simulink model "final_fuzzy"  (Simulink 10.1)
settings: Solver=ode45  StartTime=0  StopTime=1  RelTol=1e-3  EnableMultiTasking=on
libraries: powerlib x29, powerlib_extras x6, simulink x2, fuzblock x1
settings Model: Creator=kuldeep  LastModifiedBy=vardh
settings DataIOCC: LimitDataPoints=on  SignalLoggingSaveFormat=ModelDataLogs
settings OptimizationCC: ExpressionDepthLimit=2147483647
settings DebuggingCC: SolverPrmCheckMsg=warning  FcnCallInpInsideContextMsg=warning  StateNameClashWarn=warning
settings GRTTargetCC: CombineOutputUpdateFcns=on  GRTInterface=off
settings SimscapeCC: SimscapeNormalizeSystem=off

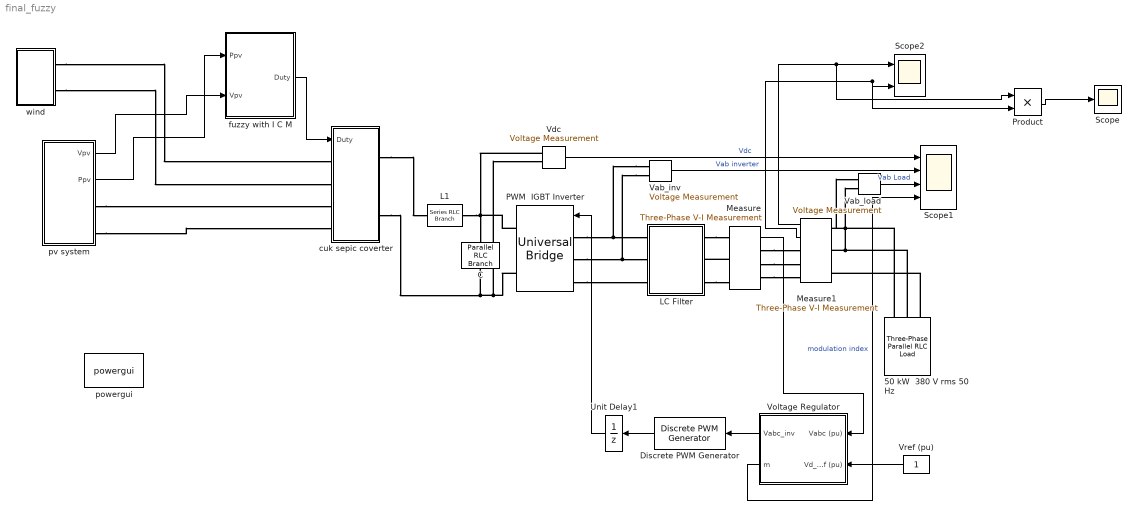
== system final_fuzzy ==
  50 kW  380 V rms 50 Hz : powerlib/Elements/Three-Phase Parallel RLC Load  LConnTagsString=A|B|C  Configuration=Y (grounded)  NominalVoltage=300  Vabc=[1e3 1e3 1e3]  Vabcp=[1e3 1e3 1e3]  NominalFrequency=50  UnbalancedPower=off  ActivePower=30e3  InductivePower=0  CapacitivePower=0  Pabc=[10e3 9e3 11e3]  QLabc=[100 90 110]  QCabc=[100 90 110]  Pabcp=[10e3 9e3 11e3]  QLabcp=[100 90 110]  QCabcp=[100 90 110]  Measurements=None  LoadType=constant Z
  C : powerlib/Elements/Parallel RLC Branch  LConnTagsString=a  RConnTagsString=__new0  BranchType=C  Resistance=inf  Inductance=inf  SetiL0=off  InitialCurrent=0  Capacitance=5000e-06  Setx0=off  InitialVoltage=0  Measurements=None
  Discrete PWM Generator : powerlib_extras/Discrete  Control Blocks/Discrete PWM Generator  GeneratorMode="3-arm  bridge (6 pulses)"  Fc=2000  Ts=3e-5  Internal=off  mIndex=0.4  Freq=60  Phase=0
      settings: SourceProductBaseCode=PS
  L1 : powerlib/Elements/Series RLC Branch  LConnTagsString=__new0  RConnTagsString=__new0  BranchType=L  Resistance=1.0  Inductance=200e-6  SetiL0=off  InitialCurrent=0  Capacitance=1.0  Setx0=off  InitialVoltage=0  Measurements=None
  LC Filter : Subsystem
  Measure : powerlib/Measurements/Three-Phase V-I Measurement  VoltageMeasurement=phase-to-ground  SetLabelV=off  LabelV=V1  Vpu=on  VpuLL=off  CurrentMeasurement=no  SetLabelI=off  LabelI=I1  Ipu=off  Pbase=1e3  Vbase=380  OutputType=Magnitude  PhasorSimulation=off  PSBequivalent=0
  Measure1 : powerlib/Measurements/Three-Phase V-I Measurement  VoltageMeasurement=phase-to-phase  SetLabelV=off  LabelV=V1  Vpu=off  VpuLL=off  CurrentMeasurement=yes  SetLabelI=off  LabelI=I1  Ipu=off  Pbase=1e3  Vbase=380  OutputType=Magnitude  PhasorSimulation=off  PSBequivalent=0
  PWM  IGBT Inverter : powerlib/Power Electronics/Universal Bridge  Arms=3  SnubberResistance=5000  SnubberCapacitance=inf  Device=IGBT / Diodes  Ron=1e-3  Lon=0  ForwardVoltages="[  0.0  0.0  ]"  ForwardVoltage=.8  GTOparameters=[ 1e-6 ,1e-6 ]  IGBTparameters=[ 1e-6 , 2e-6 ]  Measurements=Device currents  Measurements_2=None  converterType=Rectifier
  Product : Product  RndMeth=Zero
  Scope : Scope
  Scope1 : Scope  NumInputPorts=4
  Scope2 : Scope  NumInputPorts=2
  Unit Delay1 : UnitDelay  SampleTime=3e-5  HasFrameUpgradeWarning=on
  Vab_inv : powerlib/Measurements/Voltage Measurement  Tag=PoWeRsYsTeMmEaSuReMeNt  PhasorSimulation=off  OutputType=Magnitude  PSBequivalent=0
  Vab_load : powerlib/Measurements/Voltage Measurement  Tag=PoWeRsYsTeMmEaSuReMeNt  PhasorSimulation=off  OutputType=Magnitude  PSBequivalent=0
  Vdc : powerlib/Measurements/Voltage Measurement  Tag=PoWeRsYsTeMmEaSuReMeNt  PhasorSimulation=off  OutputType=Magnitude  PSBequivalent=0
  Voltage Regulator : Subsystem  mask(Voltage Regulator){Kp=0.4, Ki=500, Ts=3e-5}
      mask prompts: Kp "Proportional gain  Kp:"; Ki "Integral gain Ki:"; Ts "Sample time (s) :"
  "Vref (pu) " : Constant
  cuk sepic coverter : Subsystem
  "fuzzy with I C M " : Subsystem
  powergui : powerlib/powergui  Priority=1  SimulationMode=Discrete  SampleTime=3e-5  frequency=60  Iterations=50  frequencyindice=50  Pbase=100e6  ErrMax=1e-4  UnitsV=kV  UnitsW=MW  buscounter=0  FunctionMessages=off  echomessages=off  EnableUseOfTLC=off  CurrentSourceSwitches=off  DisableSnubberDevices=off  DisableRonSwitches=off  DisableVfSwitches=off  DisplayEquations=off  AutomaticDiscreteSolvers=off  SolverType=Tustin  Interpol=off  ExternalGateDelay=off  methode=off  Ts=100  x0status=blocks  SPID=off  SwTol=0  HookPort=off  NonlinearTolerance=1e-4  nMaxIteration=100  ContinueOnMaxIteration=off  RestoreLinks=warning  ResistiveCurrentMeasurement=off  Frange=[0:2:500]  Ylog=off  Xlog=on  ShowGrid=off  save=off  variable=ZData  structure=ScopeData12  ZoomFFT=off  StartTime=5.86  cycles=1  DisplayStyle=1  fundamental=50  FreqAxis=off  MaxFrequency=1000  frequencyindicesteady=1  RmsSteady=1  display=off
  pv system : Subsystem
  "wind " : Subsystem
  wires:
  pv system/2(Ppv) -> "fuzzy with I C M "/1(Ppv)
  pv system/1(Vpv) -> "fuzzy with I C M "/2(Vpv)
  "fuzzy with I C M "/1(Duty) -> cuk sepic coverter/1(Duty)
  "Vref (pu) "/1 -> Voltage Regulator/2(Vd_ref (pu))
  Discrete PWM Generator/1 -> Unit Delay1/1
  Voltage Regulator/1(Vabc_inv) -> Discrete PWM Generator/1
  Voltage Regulator/2(m) -> Scope1/4  "modulation index"
  Vdc/1 -> Scope1/1  "Vdc"
  Vab_load/1 -> Scope1/3  "Vab Load"
  Vab_inv/1 -> Scope1/2  "Vab inverter"
  Unit Delay1/1 -> PWM  IGBT Inverter/1
  Measure1/1 -> Scope2/1, Product/1
  Measure1/2 -> Scope2/2, Product/2
  Measure/1 -> Voltage Regulator/1(Vabc (pu))
  Product/1 -> Scope/1
  connections:
  pv system/RConn1 -- cuk sepic coverter/LConn3
  pv system/RConn2 -- cuk sepic coverter/LConn4
  "wind "/RConn1 -- cuk sepic coverter/LConn1
  "wind "/RConn2 -- cuk sepic coverter/LConn2
  PWM  IGBT Inverter/RConn2 -- Vdc/LConn2 -- C/RConn1 -- cuk sepic coverter/RConn2
  PWM  IGBT Inverter/RConn1 -- Vdc/LConn1 -- C/LConn1 -- L1/RConn1
  Vab_inv/LConn2 -- PWM  IGBT Inverter/LConn2 -- LC Filter/LConn2
  Vab_inv/LConn1 -- PWM  IGBT Inverter/LConn1 -- LC Filter/LConn1
  LC Filter/RConn1 -- Measure/LConn1
  PWM  IGBT Inverter/LConn3 -- LC Filter/LConn3
  LC Filter/RConn3 -- Measure/LConn3
  Measure/LConn2 -- LC Filter/RConn2
  cuk sepic coverter/RConn1 -- L1/LConn1
  50 kW  380 V rms 50 Hz/LConn1 -- Vab_load/LConn1 -- Measure1/LConn1
  50 kW  380 V rms 50 Hz/LConn2 -- Measure1/LConn2 -- Vab_load/LConn2
  50 kW  380 V rms 50 Hz/LConn3 -- Measure1/LConn3
  Measure/RConn1 -- Measure1/RConn1
  Measure/RConn2 -- Measure1/RConn2
  Measure/RConn3 -- Measure1/RConn3

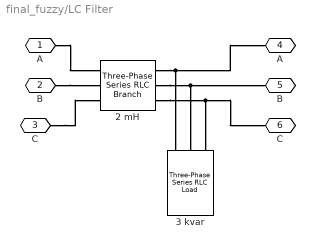
== system final_fuzzy/LC Filter ==
  "2 mH " : powerlib/Elements/Three-Phase Series RLC Branch  LConnTagsString=A|B|C  RConnTagsString=A|B|C  BranchType=L  Resistance=0  Inductance=4e-3  Capacitance=inf  Measurements=None
  3 kvar : powerlib/Elements/Three-Phase Series RLC Load  LConnTagsString=A|B|C  Configuration=Y (grounded)  NominalVoltage=380  Vabc=[1e3 1e3 1e3]  Vabcp=[1e3 1e3 1e3]  NominalFrequency=50  UnbalancedPower=off  ActivePower=0  InductivePower=0  CapacitivePower=3e-6  Pabc=[10e3 9e3 11e3]  QLabc=[100 90 110]  QCabc=[100 90 110]  Pabcp=[10e3 9e3 11e3]  QLabcp=[100 90 110]  QCabcp=[100 90 110]  Measurements=None  LoadType=constant Z
  A : PMIOPort  Side=Left
  B : PMIOPort  Port=2  Side=Left
  C : PMIOPort  Port=3  Side=Left
  "A " : PMIOPort  Port=4  Side=Right
  "B " : PMIOPort  Port=5  Side=Right
  "C " : PMIOPort  Port=6  Side=Right
  connections:
  B/RConn1 -- "2 mH "/LConn2
  A/RConn1 -- "2 mH "/LConn1
  C/RConn1 -- "2 mH "/LConn3
  "2 mH "/RConn1 -- "A "/RConn1 -- 3 kvar/LConn1
  "2 mH "/RConn2 -- "B "/RConn1 -- 3 kvar/LConn2
  "2 mH "/RConn3 -- "C "/RConn1 -- 3 kvar/LConn3

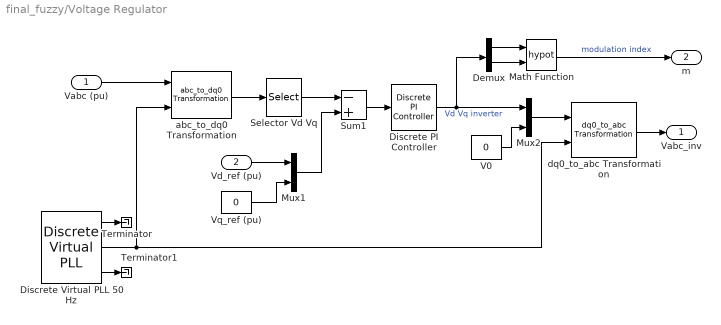
== system final_fuzzy/Voltage Regulator ==
  Vabc (pu) : Inport
  Vd_ref (pu) : Inport  Port=2
  Demux : Demux  Outputs=2
      settings: DisplayOption=none
  Discrete PI Controller : powerlib_extras/Discrete  Control Blocks/Discrete PI Controller  Kp=Kp  Ki=Ki  Par_Limits=[1 -1]  Init=0  Ts=Ts
  Discrete Virtual PLL 50 Hz : powerlib_extras/Discrete  Control Blocks/Discrete Virtual PLL  Freq=50  Phase=0  Ts=Ts
      settings: SourceProductBaseCode=PS
  Math Function : Math  Operator=hypot  SignedPower=on  SaturateOnIntegerOverflow=on
  Mux1 : Mux  Inputs=2
  Mux2 : Mux  Inputs=2
  Selector Vd Vq : Selector  InputPortWidth=3  IndexOptions=Index vector (dialog)  Indices=[1 2]  OutputSizes=1
  Sum1 : Sum  Inputs=-+  InputSameDT=on  SaturateOnIntegerOverflow=on  OutDataTypeStr=Inherit: Same as first input
  Terminator : Terminator
  Terminator1 : Terminator
  V0 : Constant  Value=0
  Vq_ref (pu) : Constant  Value=0
  abc_to_dq0 Transformation : powerlib_extras/Measurements/abc_to_dq0 Transformation
      settings: SourceProductBaseCode=PS
  dq0_to_abc Transformation : powerlib_extras/Measurements/dq0_to_abc Transformation
      settings: SourceProductBaseCode=PS
  Vabc_inv : Outport
  m : Outport  Port=2
  wires:
  abc_to_dq0 Transformation/1 -> Selector Vd Vq/1
  Vabc (pu)/1 -> abc_to_dq0 Transformation/1
  Selector Vd Vq/1 -> Sum1/1
  Sum1/1 -> Discrete PI Controller/1
  Mux2/1 -> dq0_to_abc Transformation/1
  V0/1 -> Mux2/2
  dq0_to_abc Transformation/1 -> Vabc_inv/1
  Discrete Virtual PLL 50 Hz/2 -> abc_to_dq0 Transformation/2, dq0_to_abc Transformation/2
  Vd_ref (pu)/1 -> Mux1/1
  Vq_ref (pu)/1 -> Mux1/2
  Mux1/1 -> Sum1/2
  Discrete Virtual PLL 50 Hz/1 -> Terminator/1
  Discrete Virtual PLL 50 Hz/3 -> Terminator1/1
  Discrete PI Controller/1 -> Demux/1, Mux2/1  "Vd Vq inverter"
  Demux/1 -> Math Function/1
  Demux/2 -> Math Function/2
  Math Function/1 -> m/1  "modulation index"

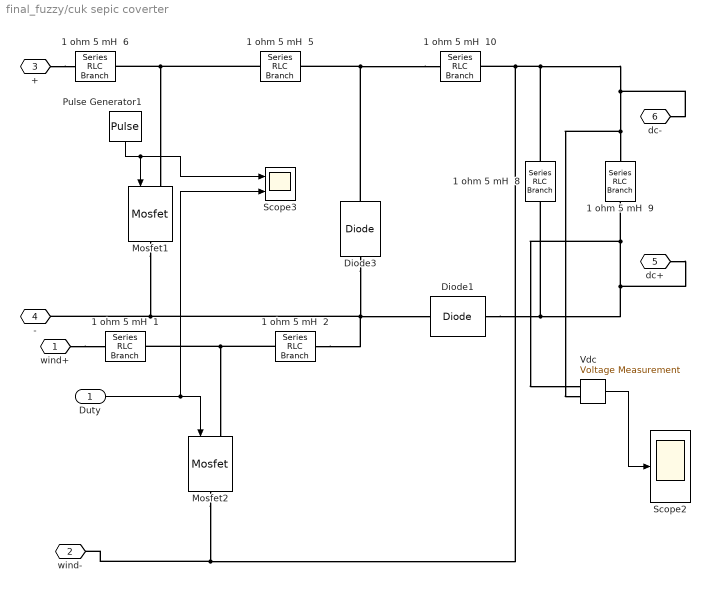
== system final_fuzzy/cuk sepic coverter ==
  Duty : Inport
  1 ohm 5 mH  1 : powerlib/Elements/Series RLC Branch  LConnTagsString=__new0  RConnTagsString=__new0  BranchType=L  Resistance=1  Inductance=2e-3  SetiL0=off  InitialCurrent=0  Capacitance=1.0  Setx0=off  InitialVoltage=0  Measurements=None
  1 ohm 5 mH  10 : powerlib/Elements/Series RLC Branch  LConnTagsString=__new0  RConnTagsString=__new0  BranchType=L  Resistance=1  Inductance=2e-3  SetiL0=off  InitialCurrent=0  Capacitance=1.0  Setx0=off  InitialVoltage=0  Measurements=None
  1 ohm 5 mH  2 : powerlib/Elements/Series RLC Branch  LConnTagsString=__new0  RConnTagsString=__new0  BranchType=C  Resistance=1  Inductance=5e-03  SetiL0=off  InitialCurrent=0  Capacitance=300e-6  Setx0=off  InitialVoltage=0  Measurements=None
  1 ohm 5 mH  5 : powerlib/Elements/Series RLC Branch  LConnTagsString=__new0  RConnTagsString=__new0  BranchType=C  Resistance=1  Inductance=5e-03  SetiL0=off  InitialCurrent=0  Capacitance=300e-6  Setx0=off  InitialVoltage=0  Measurements=None
  1 ohm 5 mH  6 : powerlib/Elements/Series RLC Branch  LConnTagsString=__new0  RConnTagsString=__new0  BranchType=L  Resistance=1  Inductance=2e-3  SetiL0=off  InitialCurrent=0  Capacitance=1.0  Setx0=off  InitialVoltage=0  Measurements=None
  1 ohm 5 mH  8 : powerlib/Elements/Series RLC Branch  LConnTagsString=__new0  RConnTagsString=__new0  BranchType=C  Resistance=1  Inductance=5e-03  SetiL0=off  InitialCurrent=0  Capacitance=5e-6  Setx0=off  InitialVoltage=0  Measurements=None
  1 ohm 5 mH  9 : powerlib/Elements/Series RLC Branch  LConnTagsString=__new0  RConnTagsString=__new0  BranchType=R  Resistance=1  Inductance=5e-03  SetiL0=off  InitialCurrent=0  Capacitance=300e-6  Setx0=off  InitialVoltage=0  Measurements=None
  Diode1 : powerlib/Power Electronics/Diode  Ron=0.001  Lon=0  Vf=0.8  IC=0  UseSnubber=off  Rs=500  Cs=250e-9  Measurements=off
  Diode3 : powerlib/Power Electronics/Diode  Ron=0.001  Lon=0  Vf=0.8  IC=0  UseSnubber=off  Rs=500  Cs=250e-9  Measurements=off
  Mosfet1 : powerlib/Power Electronics/Mosfet  Ron=0.1  Lon=0  Rd=0.01  Vfd=0  IC=0  Rs=1e5  Cs=inf  Measurements=off
  Mosfet2 : powerlib/Power Electronics/Mosfet  Ron=0.1  Lon=0  Rd=0.01  Vfd=0  IC=0  Rs=1e5  Cs=inf  Measurements=off
  Pulse Generator1 : DiscretePulseGenerator  PulseType=Time based  Period=3e-5  PulseWidth=40
  Scope2 : Scope
  Scope3 : Scope  NumInputPorts=2
  Vdc : powerlib/Measurements/Voltage Measurement  Tag=PoWeRsYsTeMmEaSuReMeNt  PhasorSimulation=off  OutputType=Magnitude  PSBequivalent=0
  wind+ : PMIOPort  Side=Left
  wind- : PMIOPort  Port=2  Side=Left
  + : PMIOPort  Port=3  Side=Left
  - : PMIOPort  Port=4  Side=Left
  dc+ : PMIOPort  Port=5  Side=Right
  dc- : PMIOPort  Port=6  Side=Right
  wires:
  Vdc/1 -> Scope2/1
  Pulse Generator1/1 -> Mosfet1/1, Scope3/1
  Duty/1 -> Mosfet2/1, Scope3/2
  connections:
  1 ohm 5 mH  1/RConn1 -- Mosfet2/LConn1 -- 1 ohm 5 mH  2/LConn1
  1 ohm 5 mH  10/LConn1 -- Diode3/LConn1 -- 1 ohm 5 mH  5/RConn1
  dc-/RConn1 -- 1 ohm 5 mH  9/RConn1 -- Vdc/LConn2 -- 1 ohm 5 mH  10/RConn1 -- Mosfet2/RConn1 -- wind-/RConn1 -- 1 ohm 5 mH  8/RConn1
  Diode3/RConn1 -- Mosfet1/RConn1 -- -/RConn1 -- 1 ohm 5 mH  2/RConn1 -- Diode1/LConn1
  1 ohm 5 mH  5/LConn1 -- 1 ohm 5 mH  6/RConn1 -- Mosfet1/LConn1
  +/RConn1 -- 1 ohm 5 mH  6/LConn1
  dc+/RConn1 -- 1 ohm 5 mH  9/LConn1 -- Vdc/LConn1 -- Diode1/RConn1 -- 1 ohm 5 mH  8/LConn1
  wind+/RConn1 -- 1 ohm 5 mH  1/LConn1

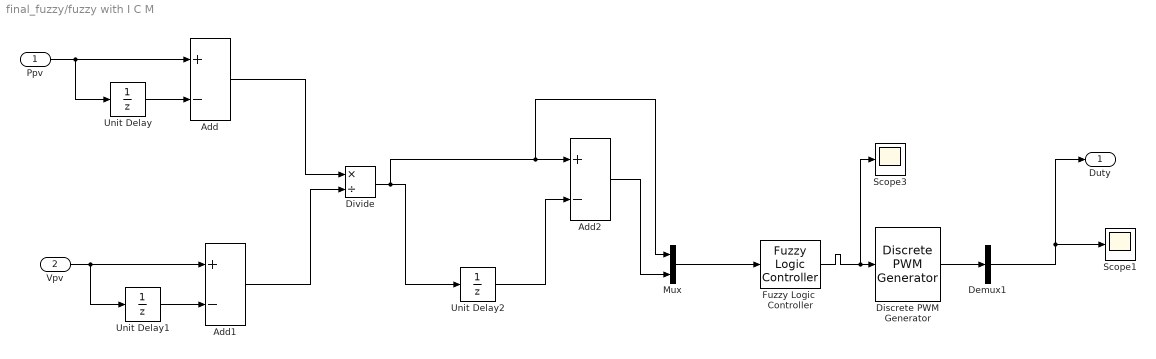
== system final_fuzzy/fuzzy with I C M  ==
  Ppv : Inport
  Vpv : Inport  Port=2
  Add : Sum  Inputs=+-
  Add1 : Sum  Inputs=+-
  Add2 : Sum  Inputs=+-
  Demux1 : Demux  Outputs=1
  Discrete PWM Generator : powerlib_extras/Discrete  Control Blocks/Discrete PWM Generator  GeneratorMode="1-arm  bridge (2 pulses)"  Fc=2000  Ts=3e-5  Internal=off  mIndex=0.4  Freq=60  Phase=0
      settings: SourceProductBaseCode=PS
  Divide : Product  Inputs=*/
  Fuzzy Logic  Controller : fuzblock/Fuzzy Logic  Controller  FIS='fuzzy_controller.fis'  OutputSampleNumber=101  DataType=double  FuzzifiedInputs=off  RuleFiringStrengths=off  RuleOutputs=off  AggregatedOutputs=off  SimulateUsing=Interpreted execution  OutOfRangeInputValueMessage=warning  NoRuleFiredMessage=warning  EmptyOutputFuzzySetMessage=warning
  Mux : Mux  Inputs=2
  Scope1 : Scope
  Scope3 : Scope
  Unit Delay : UnitDelay  SampleTime=-1  HasFrameUpgradeWarning=on
  Unit Delay1 : UnitDelay  SampleTime=-1  HasFrameUpgradeWarning=on
  Unit Delay2 : UnitDelay  SampleTime=-1  HasFrameUpgradeWarning=on
  Duty : Outport
  wires:
  Unit Delay/1 -> Add/2
  Unit Delay1/1 -> Add1/2
  Vpv/1 -> Add1/1, Unit Delay1/1
  Add/1 -> Divide/1
  Add1/1 -> Divide/2
  Add2/1 -> Mux/2
  Ppv/1 -> Unit Delay/1, Add/1
  Divide/1 -> Unit Delay2/1, Add2/1, Mux/1
  Unit Delay2/1 -> Add2/2
  Mux/1 -> Fuzzy Logic  Controller/1
  Fuzzy Logic  Controller/1 -> Discrete PWM Generator/1, Scope3/1
  Discrete PWM Generator/1 -> Demux1/1
  Demux1/1 -> Scope1/1, Duty/1

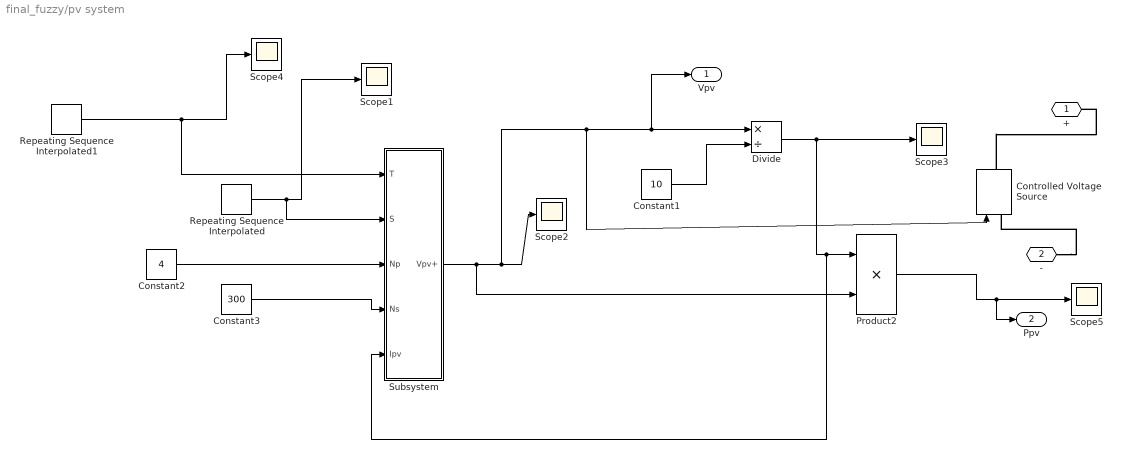
== system final_fuzzy/pv system ==
  Constant1 : Constant  Value=10
  Constant2 : Constant  Value=4
  Constant3 : Constant  Value=300
  Controlled Voltage Source : powerlib/Electrical Sources/Controlled Voltage Source  Initialize=on  Source_Type=AC  Amplitude=0  Phase=0  Frequency=0  Measurements=None
  Divide : Product  Inputs=*/
  Product2 : Product  RndMeth=Zero
  Repeating Sequence Interpolated : simulink/Sources/Repeating Sequence Interpolated  OutValues=[400 500 700 1000 700 500 400]  TimeValues=[0 1 2 3 4 5 6 ].'  LookUpMeth=Interpolation-Use End Values  tsamp=0.01  OutMin=[]  OutMax=[]  OutDataTypeStr=double  OutputDataTypeScalingMode=double  OutDataType=fixdt(0,8)  OutScaling=2^-10
  Repeating Sequence Interpolated1 : simulink/Sources/Repeating Sequence Interpolated  OutValues=[26 30 35 40 35 30 26 ].'  TimeValues=[0 1 2 3 4 5 6].'  LookUpMeth=Interpolation-Use End Values  tsamp=0.01  OutMin=[]  OutMax=[]  OutDataTypeStr=double  OutputDataTypeScalingMode=double  OutDataType=fixdt(0,8)  OutScaling=2^-10
  Scope{1..5} (5 alike) : Scope
  Subsystem : Subsystem
  + : PMIOPort  Side=Right
  - : PMIOPort  Port=2  Side=Right
  Vpv : Outport
  Ppv : Outport  Port=2
  wires:
  Repeating Sequence Interpolated1/1 -> Scope4/1, Subsystem/1(T)
  Repeating Sequence Interpolated/1 -> Scope1/1, Subsystem/2(S)
  Constant2/1 -> Subsystem/3(Np)
  Constant3/1 -> Subsystem/4(Ns)
  Subsystem/1(Vpv+) -> Scope2/1, Divide/1, Vpv/1, Controlled Voltage Source/1, Product2/2
  Constant1/1 -> Divide/2
  Divide/1 -> Scope3/1, Product2/1, Subsystem/5(Ipv)
  Product2/1 -> Scope5/1, Ppv/1
  connections:
  Controlled Voltage Source/RConn1 -- +/RConn1
  -/RConn1 -- Controlled Voltage Source/LConn1

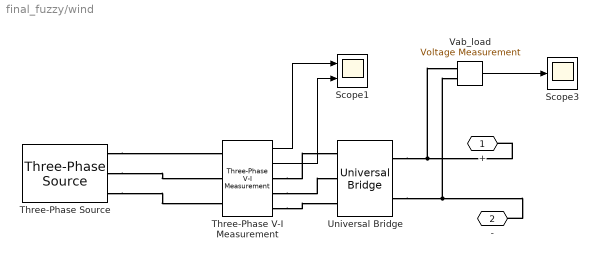
== system final_fuzzy/wind  ==
  Scope1 : Scope  NumInputPorts=2
  Scope3 : Scope
  Three-Phase V-I Measurement : powerlib/Measurements/Three-Phase V-I Measurement  VoltageMeasurement=phase-to-ground  SetLabelV=off  LabelV=Vabc  Vpu=off  VpuLL=off  CurrentMeasurement=yes  SetLabelI=off  LabelI=Iabc  Ipu=off  Pbase=100e6  Vbase=500e3  OutputType=Complex  PhasorSimulation=off  PSBequivalent=0
  Three-Phase Source : powerlib/Electrical Sources/Three-Phase Source  InternalConnection=Yg  VoltagePhases=off  Voltage=750  PhaseAngle=0  Voltage_phases=[25e3 25e3 25e3]/sqrt(3)  PhaseAngles_phases=[0 -120 +120]  Frequency=50  NonIdealSource=on  SpecifyImpedance=off  Resistance=0  Inductance=0  ShortCircuitLevel=100e6  BaseVoltage=25e3  XRratio=7  BusType=swing  Pref=0  Qref=0  Prefabc=[10e3, 10e3, 10e3]  Qrefabc=[0, 0, 0]  Qmin=-inf  Qmax=inf
  Universal Bridge : powerlib/Power Electronics/Universal Bridge  Arms=3  SnubberResistance=1e5  SnubberCapacitance=inf  Device=Diodes  Ron=1e-3  Lon=0  ForwardVoltages="[  0  0  ]"  ForwardVoltage=0  GTOparameters=[ 10e-6 , 20e-6 ]  IGBTparameters=[ 1e-6 , 2e-6 ]  Measurements=None  Measurements_2=None  converterType=Rectifier
  Vab_load : powerlib/Measurements/Voltage Measurement  Tag=PoWeRsYsTeMmEaSuReMeNt  PhasorSimulation=off  OutputType=Magnitude  PSBequivalent=0
  + : PMIOPort  Side=Right
  - : PMIOPort  Port=2  Side=Right
  wires:
  Vab_load/1 -> Scope3/1
  Three-Phase V-I Measurement/1 -> Scope1/1
  Three-Phase V-I Measurement/2 -> Scope1/2
  connections:
  Universal Bridge/RConn1 -- +/RConn1 -- Vab_load/LConn1
  Universal Bridge/RConn2 -- -/RConn1 -- Vab_load/LConn2
  Three-Phase Source/RConn1 -- Three-Phase V-I Measurement/LConn1
  Three-Phase Source/RConn2 -- Three-Phase V-I Measurement/LConn2
  Three-Phase Source/RConn3 -- Three-Phase V-I Measurement/LConn3
  Three-Phase V-I Measurement/RConn1 -- Universal Bridge/LConn1
  Three-Phase V-I Measurement/RConn2 -- Universal Bridge/LConn2
  Three-Phase V-I Measurement/RConn3 -- Universal Bridge/LConn3

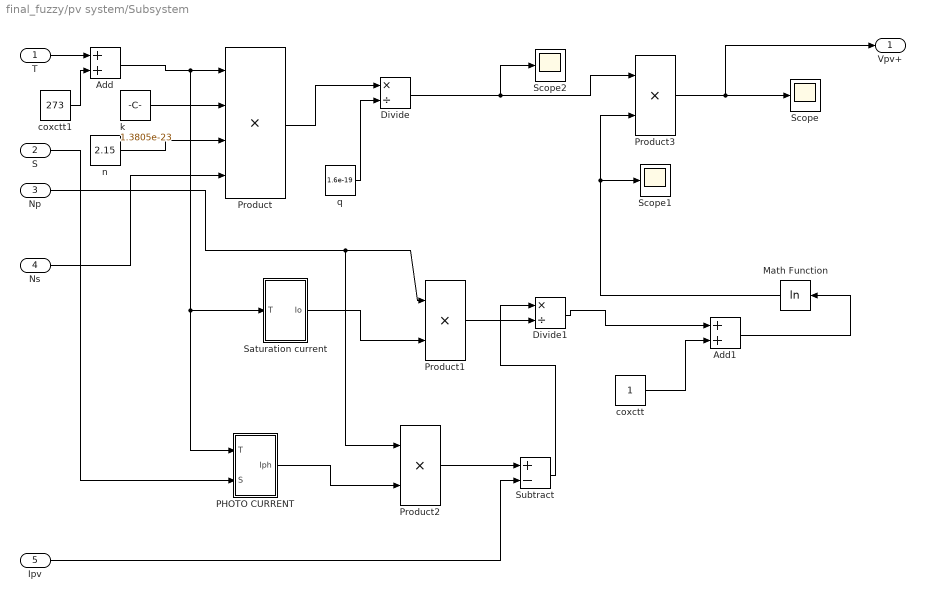
== system final_fuzzy/pv system/Subsystem ==
  T : Inport
  S : Inport  Port=2
  Np : Inport  Port=3
  Ns : Inport  Port=4
  Ipv : Inport  Port=5
  Add : Sum
  Add1 : Sum
  Divide : Product  Inputs=*/
  Divide1 : Product  Inputs=*/
  Math Function : Math  Operator=log  SignedPower=on  SaturateOnIntegerOverflow=on
  PHOTO CURRENT : Subsystem
  Product : Product  Inputs=4  RndMeth=Zero
  Product1 : Product  RndMeth=Zero
  Product2 : Product  RndMeth=Zero
  Product3 : Product  RndMeth=Zero
  Saturation current : Subsystem
  Scope : Scope
  Scope1 : Scope
  Scope2 : Scope
  Subtract : Sum  Inputs=+-
  coxctt : Constant
  coxctt1 : Constant  Value=273
  k : Constant  Value=1.3805e-23
  n : Constant  Value=2.15
  q : Constant  Value=1.6e-19
  Vpv+ : Outport
  wires:
  T/1 -> Add/1
  Add/1 -> Product/1, PHOTO CURRENT/1(T), Saturation current/1(T)
  Ns/1 -> Product/4
  n/1 -> Product/3
  k/1 -> Product/2
  Product/1 -> Divide/1
  q/1 -> Divide/2
  S/1 -> PHOTO CURRENT/2(S)
  Np/1 -> Product2/1, Product1/1
  Saturation current/1(Io) -> Product1/2
  PHOTO CURRENT/1(Iph) -> Product2/2
  Product2/1 -> Subtract/1
  Subtract/1 -> Divide1/1
  Product1/1 -> Divide1/2
  Divide1/1 -> Add1/1
  coxctt/1 -> Add1/2
  Add1/1 -> Math Function/1
  Divide/1 -> Product3/1, Scope2/1
  Math Function/1 -> Product3/2, Scope1/1
  coxctt1/1 -> Add/2
  Ipv/1 -> Subtract/2
  Product3/1 -> Scope/1, Vpv+/1

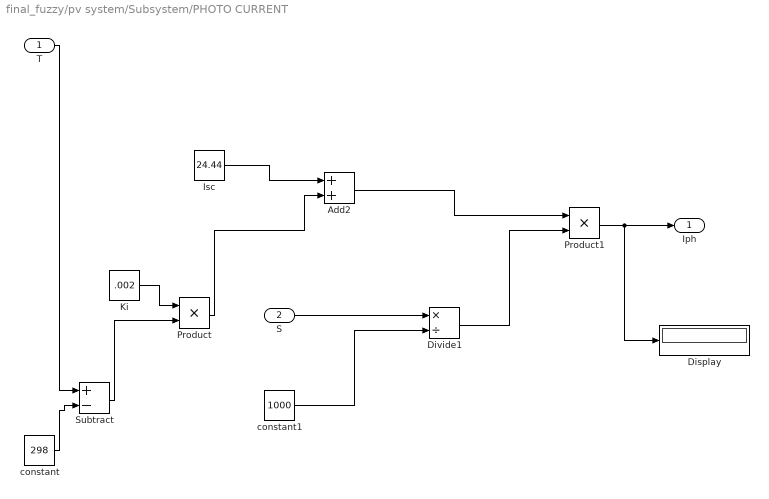
== system final_fuzzy/pv system/Subsystem/PHOTO CURRENT ==
  T : Inport
  S : Inport  Port=2
  Add2 : Sum
  Display : Display
  Divide1 : Product  Inputs=*/
  Isc : Constant  Value=24.44
  Ki : Constant  Value=.002
  Product : Product  RndMeth=Zero
  Product1 : Product  RndMeth=Zero
  Subtract : Sum  Inputs=+-
  constant : Constant  Value=298
  constant1 : Constant  Value=1000
  Iph : Outport
  wires:
  T/1 -> Subtract/1
  Isc/1 -> Add2/1
  Ki/1 -> Product/1
  constant/1 -> Subtract/2
  Subtract/1 -> Product/2
  Product/1 -> Add2/2
  Divide1/1 -> Product1/2
  Add2/1 -> Product1/1
  Product1/1 -> Iph/1, Display/1
  S/1 -> Divide1/1
  constant1/1 -> Divide1/2

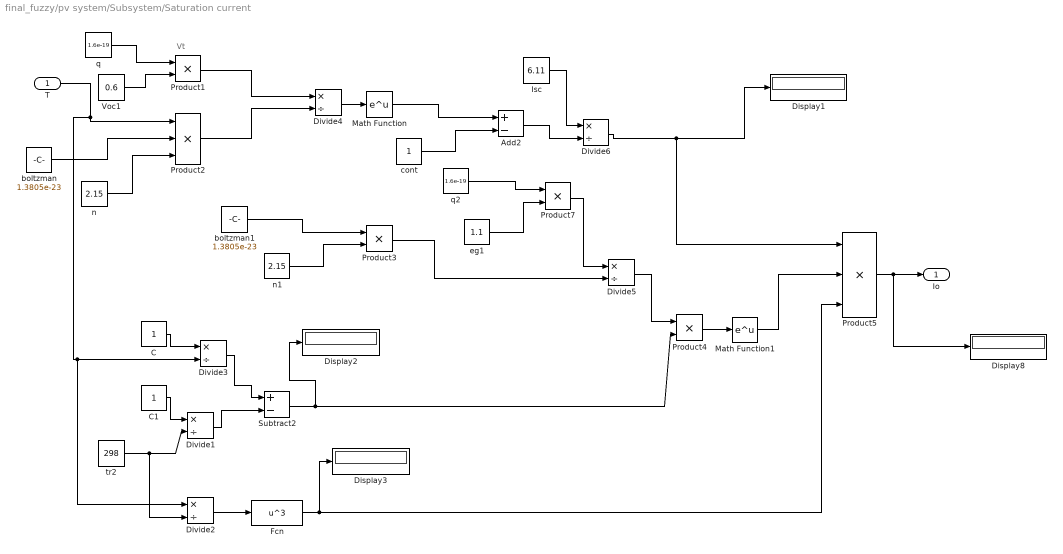
== system final_fuzzy/pv system/Subsystem/Saturation current ==
  note: Vt
  T : Inport
  Add2 : Sum  Inputs=+-
  C : Constant
  C1 : Constant
  Display{1..3,8} (4 alike) : Display
  Divide{1..6} (6 alike) : Product  Inputs=*/
  Fcn : Fcn  Expr=u^3
  Isc : Constant  Value=6.11
  Math Function : Math  SignedPower=on  SaturateOnIntegerOverflow=on
  Math Function1 : Math  SignedPower=on  SaturateOnIntegerOverflow=on
  Product{1,3..4,7} (4 alike) : Product  RndMeth=Zero
  Product2 : Product  Inputs=3  RndMeth=Zero
  Product5 : Product  Inputs=3  RndMeth=Zero
  Subtract2 : Sum  Inputs=+-
  Voc1 : Constant  Value=0.6
  boltzman : Constant  Value=1.3805e-23
  boltzman1 : Constant  Value=1.3805e-23
  cont : Constant
  eg1 : Constant  Value=1.1
  n : Constant  Value=2.15
  n1 : Constant  Value=2.15
  q : Constant  Value=1.6e-19
  q2 : Constant  Value=1.6e-19
  tr2 : Constant  Value=298
  Io : Outport
  wires:
  Isc/1 -> Divide6/1
  Divide6/1 -> Display1/1, Product5/1
  q/1 -> Product1/1
  boltzman/1 -> Product2/2
  n/1 -> Product2/3
  Product1/1 -> Divide4/1
  Product2/1 -> Divide4/2
  Add2/1 -> Divide6/2
  Voc1/1 -> Product1/2
  Divide4/1 -> Math Function/1
  Math Function/1 -> Add2/1
  cont/1 -> Add2/2
  tr2/1 -> Divide1/2, Divide2/2
  C/1 -> Divide3/1
  C1/1 -> Divide1/1
  Divide1/1 -> Subtract2/2
  Divide3/1 -> Subtract2/1
  Subtract2/1 -> Display2/1, Product4/2
  Divide2/1 -> Fcn/1
  Fcn/1 -> Display3/1, Product5/3
  boltzman1/1 -> Product3/1
  n1/1 -> Product3/2
  q2/1 -> Product7/1
  eg1/1 -> Product7/2
  Product7/1 -> Divide5/1
  Product3/1 -> Divide5/2
  Divide5/1 -> Product4/1
  Product4/1 -> Math Function1/1
  Math Function1/1 -> Product5/2
  Product5/1 -> Io/1, Display8/1
  T/1 -> Product2/1, Divide3/2, Divide2/1
